simulink model "subsistema_electromagnetico2"  (R2023b)
settings: Solver=VariableStepAuto  StartTime=0.0  StopTime=10.0  RelTol=1e-3
values from neighbouring files (symbols this model uses):
  L_d = 6.6    [analisis_estabilidad.m]    (also in parametros.m = 0.0066; parametros_sim.m; polosyceros.m = L_d^3)
  L_ls = 0.8    [analisis_estabilidad.m]    (also in parametros.m = 0.0008; parametros_sim.m)
  L_q = 5.8    [analisis_estabilidad.m]    (also in parametros.m = 0.0058; parametros_sim.m; polosyceros.m = L_q^3)
  lambda_m = 0.016    [analisis_estabilidad.m]    (also in parametros.m; parametros_sim.m)
  P_p = 3    [analisis_estabilidad.m]    (also in parametros.m; parametros_sim.m)
settings Model: Creator=Marti  LastModifiedBy=Marti

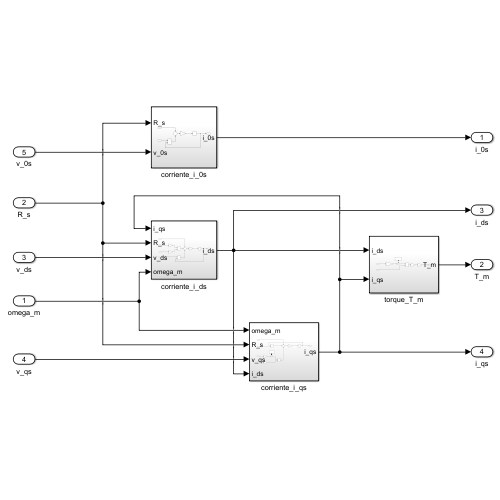
[thumbnail: Simulink's stored preview of the top-level diagram]
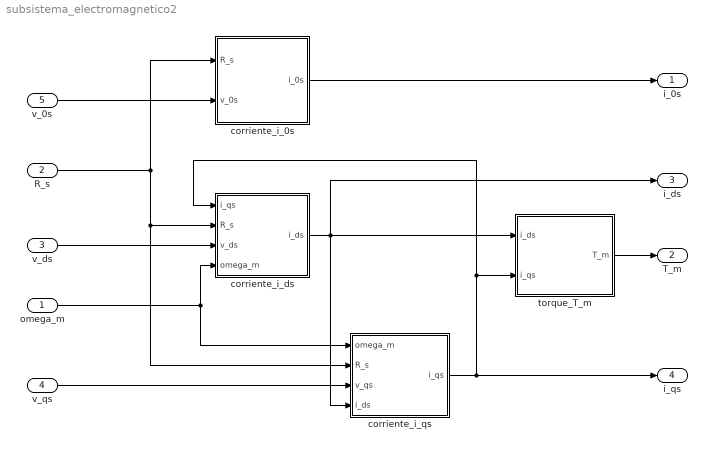
== system subsistema_electromagnetico2 ==
  omega_m : Inport
  R_s : Inport  Port=2
  v_ds : Inport  Port=3
  v_qs : Inport  Port=4
  v_0s : Inport  Port=5
  corriente_i_0s : Subsystem
  corriente_i_ds : Subsystem
  corriente_i_qs : Subsystem
  torque_T_m : Subsystem
  i_0s : Outport
  T_m : Outport  Port=2
  i_ds : Outport  Port=3
  i_qs : Outport  Port=4
  wires:
  omega_m/1 -> corriente_i_qs/1(omega_m), corriente_i_ds/4(omega_m)
  corriente_i_ds/1(i_ds) -> i_ds/1, torque_T_m/1(i_ds), corriente_i_qs/4(i_ds)
  corriente_i_qs/1(i_qs) -> torque_T_m/2(i_qs), corriente_i_ds/1(i_qs), i_qs/1
  R_s/1 -> corriente_i_0s/1(R_s), corriente_i_qs/2(R_s), corriente_i_ds/2(R_s)
  v_ds/1 -> corriente_i_ds/3(v_ds)
  v_qs/1 -> corriente_i_qs/3(v_qs)
  v_0s/1 -> corriente_i_0s/2(v_0s)
  corriente_i_0s/1(i_0s) -> i_0s/1
  torque_T_m/1(T_m) -> T_m/1

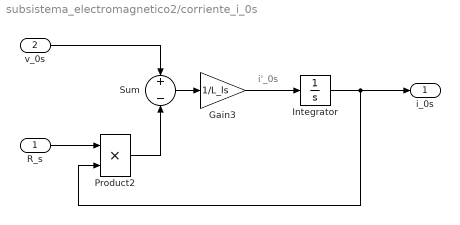
== system subsistema_electromagnetico2/corriente_i_0s ==
  note: i'_0s
  R_s : Inport
  v_0s : Inport  Port=2
  Gain3 : Gain  Gain=1/L_ls
  Integrator : Integrator
  Product2 : Product
  Sum : Sum  Inputs=+-
  i_0s : Outport
  wires:
  Integrator/1 -> i_0s/1, Product2/2
  Sum/1 -> Gain3/1
  v_0s/1 -> Sum/1
  Gain3/1 -> Integrator/1
  Product2/1 -> Sum/2
  R_s/1 -> Product2/1

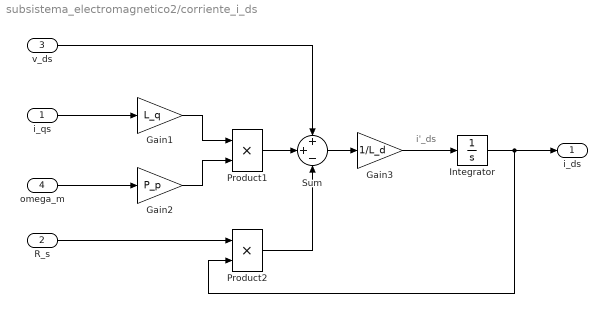
== system subsistema_electromagnetico2/corriente_i_ds ==
  note: i'_ds
  i_qs : Inport
  R_s : Inport  Port=2
  v_ds : Inport  Port=3
  omega_m : Inport  Port=4
  Gain1 : Gain  Gain=L_q
  Gain2 : Gain  Gain=P_p
  Gain3 : Gain  Gain=1/L_d
  Integrator : Integrator
  Product1 : Product
  Product2 : Product
  Sum : Sum  Inputs=++-
  i_ds : Outport
  wires:
  Product1/1 -> Sum/2
  omega_m/1 -> Gain2/1
  Gain1/1 -> Product1/1
  Gain2/1 -> Product1/2
  Gain3/1 -> Integrator/1
  i_qs/1 -> Gain1/1
  v_ds/1 -> Sum/1
  Integrator/1 -> i_ds/1, Product2/2
  Product2/1 -> Sum/3
  Sum/1 -> Gain3/1
  R_s/1 -> Product2/1

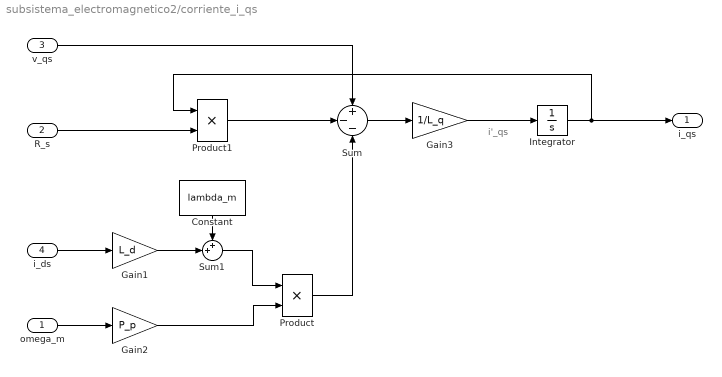
== system subsistema_electromagnetico2/corriente_i_qs ==
  note: i'_qs
  omega_m : Inport
  R_s : Inport  Port=2
  v_qs : Inport  Port=3
  i_ds : Inport  Port=4
  Constant : Constant  Value=lambda_m
  Gain1 : Gain  Gain=L_d
  Gain2 : Gain  Gain=P_p
  Gain3 : Gain  Gain=1/L_q
  Integrator : Integrator
  Product : Product
  Product1 : Product
  Sum : Sum  Inputs=+--
  Sum1 : Sum  Inputs=++|
  i_qs : Outport
  wires:
  Constant/1 -> Sum1/1
  Gain1/1 -> Sum1/2
  Integrator/1 -> i_qs/1, Product1/1
  v_qs/1 -> Sum/1
  Product/1 -> Sum/3
  Sum1/1 -> Product/1
  Sum/1 -> Gain3/1
  i_ds/1 -> Gain1/1
  omega_m/1 -> Gain2/1
  Gain3/1 -> Integrator/1
  Product1/1 -> Sum/2
  Gain2/1 -> Product/2
  R_s/1 -> Product1/2

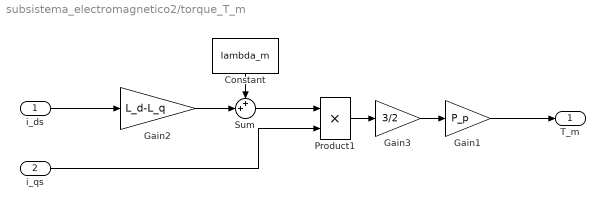
== system subsistema_electromagnetico2/torque_T_m ==
  i_ds : Inport
  i_qs : Inport  Port=2
  Constant : Constant  Value=lambda_m
  Gain1 : Gain  Gain=P_p
  Gain2 : Gain  Gain=L_d-L_q
  Gain3 : Gain  Gain=3/2
  Product1 : Product
  Sum : Sum  Inputs=++|
  T_m : Outport
  wires:
  i_ds/1 -> Gain2/1
  Gain2/1 -> Sum/2
  Product1/1 -> Gain3/1
  Sum/1 -> Product1/1
  Constant/1 -> Sum/1
  i_qs/1 -> Product1/2
  Gain3/1 -> Gain1/1
  Gain1/1 -> T_m/1
